simulink model "DCmotor"  (R2014b)
settings: Solver=ode45  StartTime=0.0  StopTime=10.0  RelTol=1e-3
values from neighbouring files (symbols this model uses):
  Cv = 1.3*10^(-3) *10^(-3) *60    (= 7.8e-05)    [load_values.m]    (also in task6.m = 1.24140855612e-05)
  J = 60 * 10^(-3) *10^(-4)    (= 6e-06)    [load_values.m]    (also in task6.m)
  kE = 4.555 *10^(-3) *60    (= 0.2733)    [load_values.m]    (also in task6.m = 0.043497045947)
  kM = 43.5*10^(-3)    (= 0.0435)    [load_values.m]    (also in task6.m)
  L = 110*10^(-6)    (= 0.00011)    [load_values.m]    (also in task6.m)
  R = 1.45    [load_values.m]    (also in task6.m)
settings Model: Creator=Davide  LastModifiedBy=Davide
settings DebuggingCC: SolverPrmCheckMsg=none

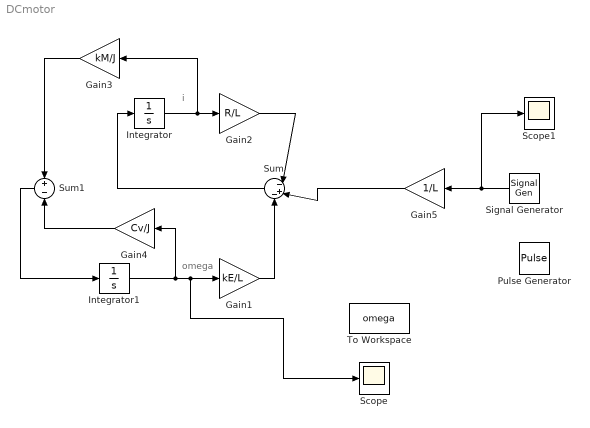
== system DCmotor ==
  note: omega
  note: i
  Gain1 : Gain  Gain=kE/L
  Gain2 : Gain  Gain=R/L
  Gain3 : Gain  Gain=kM/J
  Gain4 : Gain  Gain=Cv/J
  Gain5 : Gain  Gain=1/L
  Integrator : Integrator
  Integrator1 : Integrator
  Pulse Generator : DiscretePulseGenerator  PulseType=Time based  Amplitude=24  Period=10  PulseWidth=10
  Scope : Scope
      settings: TimeRange=10
  Scope1 : Scope
      settings: TimeRange=10
  Signal Generator : SignalGenerator  WaveForm=square  Frequency=0.1
  Sum : Sum  Inputs=|-+-
  Sum1 : Sum  Inputs=+|-
  To Workspace : ToWorkspace  VariableName=omega  SaveFormat=Timeseries  SampleTime=-1
  wires:
  Integrator/1 -> Gain3/1, Gain2/1
  Integrator1/1 -> Gain4/1, Scope/1, Gain1/1
  Gain2/1 -> Sum/1
  Sum/1 -> Integrator/1
  Gain1/1 -> Sum/3
  Gain3/1 -> Sum1/1
  Gain4/1 -> Sum1/2
  Sum1/1 -> Integrator1/1
  Gain5/1 -> Sum/2
  Signal Generator/1 -> Scope1/1, Gain5/1
